simulink library "INT_CoPT_ThermDem"  (R2016b)
settings: Solver=VariableStepAuto  StartTime=0.0  StopTime=10.0  RelTol=1e-3
settings Model: Creator=bianxuyin  LastModifiedBy=bianxuyin

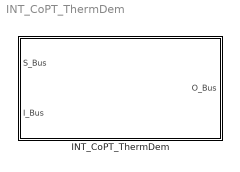
== system INT_CoPT_ThermDem ==
  INT_CoPT_ThermDem : Subsystem

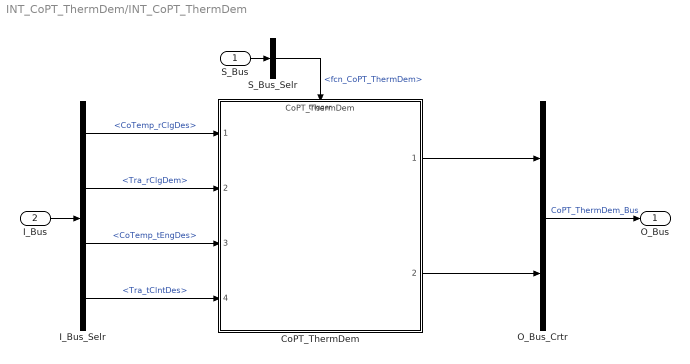
== system INT_CoPT_ThermDem/INT_CoPT_ThermDem ==
  S_Bus : Inport
  I_Bus : Inport  Port=2
  CoPT_ThermDem : ModelReference  ModelNameDialog=CoPT_ThermDem  SimulationMode=Normal  ModelReferenceVersion=1.7  TriggerPortName=function  TriggerPortTriggerType=function-call  TriggerPortStatesWhenEnabling=held
  I_Bus_Selr : BusSelector  OutputSignals=CoTemp_rClgDes,Tra_rClgDem,CoTemp_tEngDes,Tra_tClntDes
  O_Bus_Crtr : BusCreator  Inputs=2
  S_Bus_Selr : BusSelector  OutputSignals=fcn_CoPT_ThermDem
  O_Bus : Outport
  wires:
  S_Bus_Selr/1 -> CoPT_ThermDem/Trigger  "<fcn_CoPT_ThermDem>"
  S_Bus/1 -> S_Bus_Selr/1
  I_Bus/1 -> I_Bus_Selr/1
  I_Bus_Selr/1 -> CoPT_ThermDem/1  "<CoTemp_rClgDes>"
  I_Bus_Selr/2 -> CoPT_ThermDem/2  "<Tra_rClgDem>"
  I_Bus_Selr/3 -> CoPT_ThermDem/3  "<CoTemp_tEngDes>"
  I_Bus_Selr/4 -> CoPT_ThermDem/4  "<Tra_tClntDes>"
  O_Bus_Crtr/1 -> O_Bus/1  "CoPT_ThermDem_Bus"
  CoPT_ThermDem/1 -> O_Bus_Crtr/1
  CoPT_ThermDem/2 -> O_Bus_Crtr/2
